simulink model "buck"  (R2020b)
settings: Solver=VariableStepAuto  StartTime=0.0  StopTime=2  RelTol=1e-3
libraries: powerlib x12
settings Model: Creator=shashank Pathak  LastModifiedBy=shashank Pathak

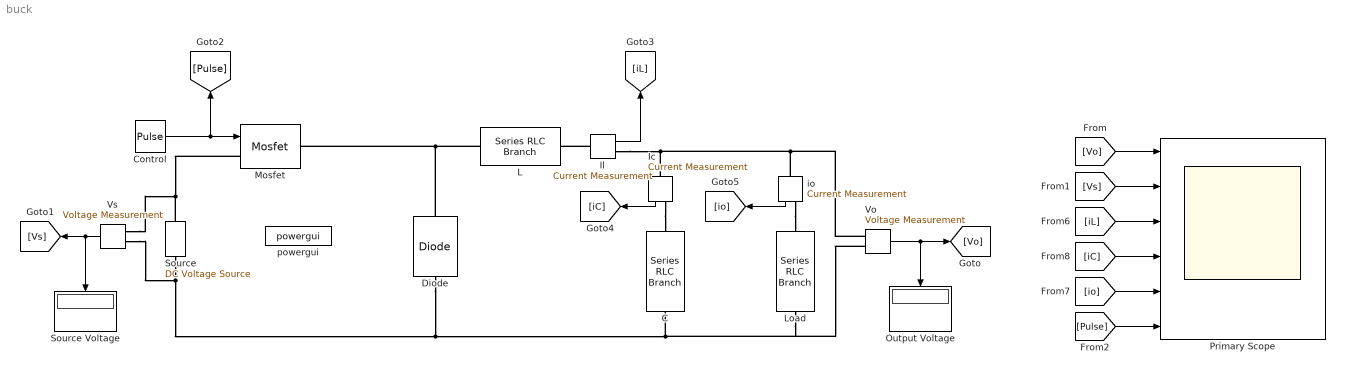
== system buck ==
  C : powerlib/Elements/Series RLC Branch  LConnTagsString=__new0  RConnTagsString=__new0  BranchType=C  Resistance=1  Inductance=1e-3  SetiL0=off  InitialCurrent=0  Capacitance=220e-6  Setx0=off  InitialVoltage=0  Measurements=None
  Control : DiscretePulseGenerator  PulseType=Time based  Period=1/10000  PulseWidth=50
  Diode : powerlib/Power Electronics/Diode  Ron=0  Lon=0  Vf=0  IC=0  UseSnubber=0  Rs=0  Cs=0  Measurements=off
  Ic : powerlib/Measurements/Current Measurement  PhasorSimulation=off  OutputType=Complex  PSBequivalent=0
  Il : powerlib/Measurements/Current Measurement  PhasorSimulation=off  OutputType=Complex  PSBequivalent=0
  L : powerlib/Elements/Series RLC Branch  LConnTagsString=__new0  RConnTagsString=__new0  BranchType=L  Resistance=1  Inductance=5e-3  SetiL0=off  InitialCurrent=0  Capacitance=1e-6  Setx0=off  InitialVoltage=0  Measurements=None
  Load : powerlib/Elements/Series RLC Branch  LConnTagsString=__new0  RConnTagsString=__new0  BranchType=R  Resistance=10  Inductance=1e-3  SetiL0=off  InitialCurrent=0  Capacitance=1e-6  Setx0=off  InitialVoltage=0  Measurements=None
  Mosfet : powerlib/Power Electronics/Mosfet  Ron=0  Lon=0.0000001  Rd=0  Vfd=0  IC=0  Rs=1e5  Cs=inf  Measurements=off
  Output Voltage : Display
  Primary Scope : Scope  NumInputPorts=6
  Source : powerlib/Electrical Sources/DC Voltage Source  Amplitude=100  Measurements=None
  Source Voltage : Display
  Vo : powerlib/Measurements/Voltage Measurement  PhasorSimulation=off  OutputType=Complex  PSBequivalent=0
  Vs : powerlib/Measurements/Voltage Measurement  PhasorSimulation=off  OutputType=Complex  PSBequivalent=0
  io : powerlib/Measurements/Current Measurement  PhasorSimulation=off  OutputType=Complex  PSBequivalent=0
  powergui : powerlib/powergui  Priority=1  SimulationMode=Continuous  SampleTime=50e-6  frequency=60  Iterations=50  frequencyindice=0  Pbase=100e6  ErrMax=1e-4  UnitsV=kV  UnitsW=MW  buscounter=0  FunctionMessages=off  echomessages=off  EnableUseOfTLC=off  CurrentSourceSwitches=off  DisableSnubberDevices=off  DisableRonSwitches=off  DisableVfSwitches=off  DisplayEquations=off  AutomaticDiscreteSolvers=off  SolverType=Tustin/Backward Euler (TBE)  Interpol=off  ExternalGateDelay=off  methode=off  Ts=100  x0status=blocks  SPID=on  SwTol=0  HookPort=off  NonlinearTolerance=1e-4  nMaxIteration=100  ContinueOnMaxIteration=off  RestoreLinks=warning  ResistiveCurrentMeasurement=off  Frange=[0:2:500]  Ylog=off  Xlog=on  ShowGrid=off  save=off  variable=ZData  structure=0  ZoomFFT=off  StartTime=0.0  cycles=1  DisplayStyle=1  fundamental=60  FreqAxis=off  MaxFrequency=1000  frequencyindicesteady=1  RmsSteady=1  display=off
  wires:
  Vo/1 -> [Vo], Output Voltage/1
  Vs/1 -> [Vs], Source Voltage/1
  Control/1 -> [Pulse], Mosfet/1
  Il/1 -> [iL]
  Ic/1 -> [iC]
  io/1 -> [io]
  [Vo] -> Primary Scope/1
  [iL] -> Primary Scope/3
  [iC] -> Primary Scope/4
  [Pulse] -> Primary Scope/6
  [io] -> Primary Scope/5
  [Vs] -> Primary Scope/2
  connections:
  Source/RConn1 -- Mosfet/LConn1 -- Vs/LConn1
  L/LConn1 -- Diode/RConn1 -- Mosfet/RConn1
  Source/LConn1 -- Vs/LConn2 -- C/RConn1 -- Load/RConn1 -- Vo/LConn2 -- Diode/LConn1
  Il/LConn1 -- L/RConn1
  Ic/RConn1 -- C/LConn1
  io/RConn1 -- Load/LConn1
  Vo/LConn1 -- Il/RConn1 -- Ic/LConn1 -- io/LConn1
